simulink model "M_ZH_Z4"  (R2025a)
settings: Solver=VariableStepAuto  StartTime=0.0  StopTime=20e-3  MaxStep=560*33e-9/25  RelTol=1e-3
libraries: simulink_extras x1
settings Model: Creator=Szalay  LastModifiedBy=Szalay

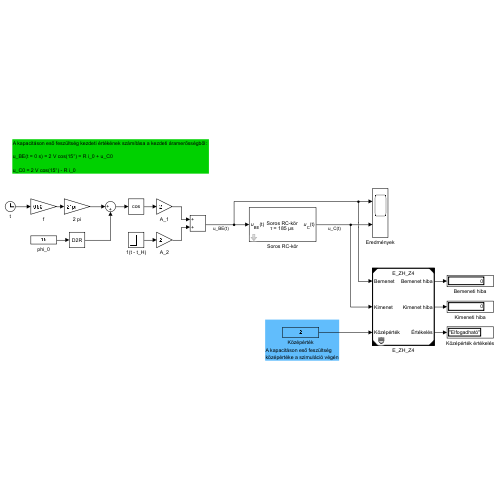
[thumbnail: Simulink's stored preview of the top-level diagram]
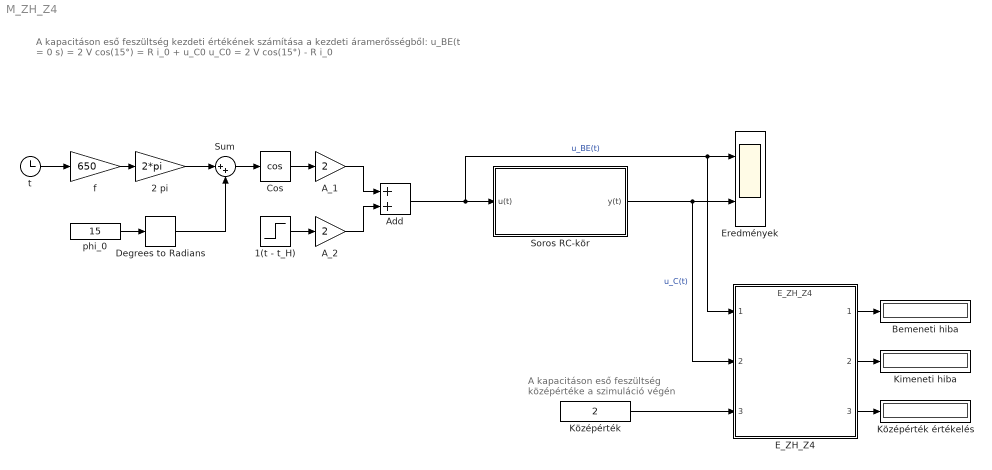
== system M_ZH_Z4 ==
  note: A kapacitáson eső feszültség kezdeti értékének számítása a kezdeti áramerősségből:
      |
      | u_BE(t = 0 s) = 2 V cos(15°) = R i_0 + u_C0
      |
      | u_C0 = 2 V cos(15°) - R i_0
  note: A kapacitáson eső feszültség
      | középértéke a szimuláció végén
  1(t - t_H) : Step  Time=10e-3  SampleTime=0
  2 pi : Gain  Gain=2*pi
  A_1 : Gain  Gain=2
  A_2 : Gain  Gain=2
  Add : Sum
  Bemeneti hiba : Display
  Cos : Trigonometry  Operator=cos
  Degrees to Radians : simulink_extras/Transformations/Degrees to Radians
  E_ZH_Z4 : ModelReference  ModelNameDialog=E_ZH_Z4.slxp  ModelReferenceVersion=1.10  CopyOfModelProtected=on
  Eredmények : Scope  NumInputPorts=2
      settings: ActiveDisplayYMinimum=-4.6266668908158941  ActiveDisplayYMaximum=4.9585185431244128
  Kimeneti hiba : Display
  Középérték : Constant  Value=2
  Középérték értékelés : Display
  Soros RC-kör : Subsystem  mask(Soros RC-kör){R=5600, C=33e-9, u_C0=2*cos(deg2rad(15)) - 5600*1e-3}
      mask prompts: R "Ellenállás (Ohm)"; C "Kapacitás (F)"; u_C0 "A kapacitás kezdeti feszültsége"
      mask help: A soros RC-kör modellje.
      mask DialogControl ParameterGroupVar Prompt: Rendszerparaméterek
      mask DialogControl Container3 Prompt: Kezdeti érték
      mask Display:
      | % Csatlakozók
      | port_label('input', 1, '{\itu}_{BE}(t)', 'texmode', 'on');
      | port_label('output', 1, '{\itu}_C(t)', 'texmode', 'on');
      | 
      | R = str2double(get_param(gcb, 'R'));
      | C = str2double(get_param(gcb, 'C'));
      | 
      | % Felirat
      | text(0.5, 0.5, ...
      |     sprintf('Soros RC-kör\n\\tau = %.3g \\mus', 1e6*R*C), ...
      |     'HorizontalAlignment', 'center', ...
      |     'Interpreter', 'tex' ...
      |     );
  Sum : Sum  Inputs=|++
  f : Gain  Gain=650
  phi_0 : Constant  Value=15
  t : Clock
  wires:
  A_1/1 -> Add/1
  A_2/1 -> Add/2
  Cos/1 -> A_1/1
  1(t - t_H)/1 -> A_2/1
  t/1 -> f/1
  2 pi/1 -> Sum/1
  f/1 -> 2 pi/1
  Sum/1 -> Cos/1
  phi_0/1 -> Degrees to Radians/1
  Degrees to Radians/1 -> Sum/2
  Add/1 -> E_ZH_Z4/1, Eredmények/1, Soros RC-kör/1(u(t))  "u_BE(t)"
  Soros RC-kör/1(y(t)) -> E_ZH_Z4/2, Eredmények/2  "u_C(t)"
  Középérték/1 -> E_ZH_Z4/3
  E_ZH_Z4/3 -> Középérték értékelés/1
  E_ZH_Z4/2 -> Kimeneti hiba/1
  E_ZH_Z4/1 -> Bemeneti hiba/1

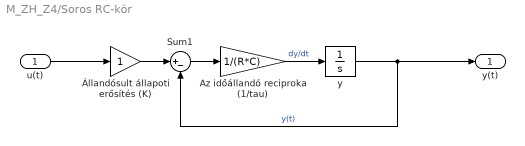
== system M_ZH_Z4/Soros RC-kör ==
  u(t) : Inport
  Az időállandó reciproka (1/tau) : Gain  Gain=1/(R*C)
  Sum1 : Sum  Inputs=|+-
  y : Integrator  InitialCondition=u_C0
  Állandósult állapoti erősítés (K) : Gain
  y(t) : Outport
  wires:
  Az időállandó reciproka (1/tau)/1 -> y/1  "dy/dt"
  Sum1/1 -> Az időállandó reciproka (1/tau)/1
  y/1 -> y(t)/1, Sum1/2  "y(t)"
  Állandósult állapoti erősítés (K)/1 -> Sum1/1
  u(t)/1 -> Állandósult állapoti erősítés (K)/1
